simulink model "lab2p2"  (R2022a)
settings: Solver=VariableStepAuto  StartTime=0.0  StopTime=20  RelTol=1e-3
settings Model: Creator=tylergs2  LastModifiedBy=tylergs2

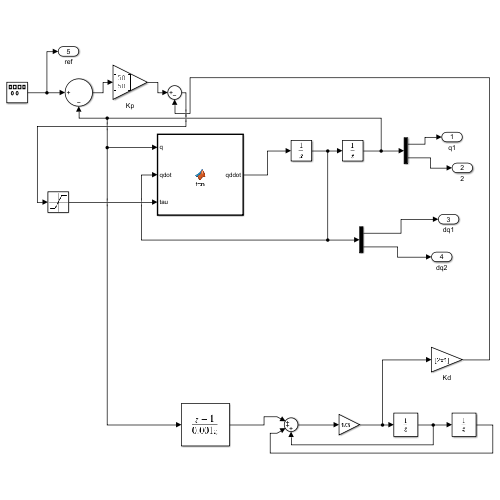
[thumbnail: Simulink's stored preview of the top-level diagram]
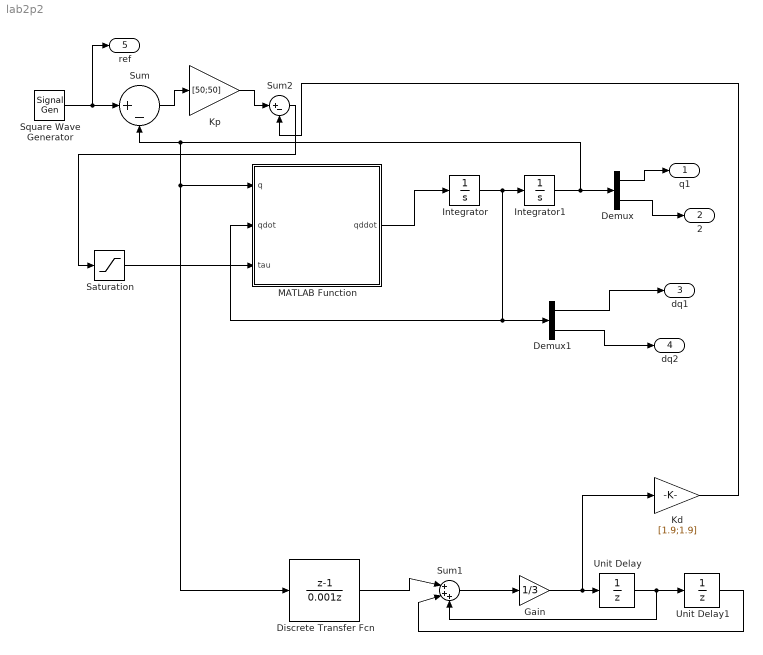
== system lab2p2 ==
  Demux : Demux  Outputs=2
  Demux1 : Demux  Outputs=2
  Discrete Transfer Fcn : DiscreteTransferFcn  Numerator="[1  -1]"  Denominator=[0.001 0]  SampleTime=0.001
  Gain : Gain  Gain=1/3
  Integrator : Integrator  InitialCondition=[0;0]
  Integrator1 : Integrator  InitialCondition=[0;0]
  Kd : Gain  Gain=[1.9;1.9]
  Kp : Gain  Gain=[50;50]
  MATLAB Function : MATLAB Function  TreatAsAtomicUnit=on
  Saturation : Saturate  UpperLimit=5  LowerLimit=-5
  Square Wave Generator : SignalGenerator  WaveForm=square  Amplitude=0.25  Frequency=0.25
  Sum : Sum  Inputs=|+-
  Sum1 : Sum  Inputs=|+++
  Sum2 : Sum  Inputs=|+-
  Unit Delay : UnitDelay  SampleTime=0.001  HasFrameUpgradeWarning=on
  Unit Delay1 : UnitDelay  SampleTime=0.001  HasFrameUpgradeWarning=on
  q1 : Outport
  2 : Outport  Port=2
  dq1 : Outport  Port=3
  dq2 : Outport  Port=4
  ref : Outport  Port=5
  wires:
  MATLAB Function/1(qddot) -> Integrator/1
  Integrator/1 -> Demux1/1, MATLAB Function/2(qdot), Integrator1/1
  Sum/1 -> Kp/1
  Discrete Transfer Fcn/1 -> Sum1/1
  Unit Delay1/1 -> Sum1/2
  Integrator1/1 -> Sum/2, Discrete Transfer Fcn/1, MATLAB Function/1(q), Demux/1
  Unit Delay/1 -> Sum1/3, Unit Delay1/1
  Gain/1 -> Kd/1, Unit Delay/1
  Sum1/1 -> Gain/1
  Kp/1 -> Sum2/1
  Kd/1 -> Sum2/2
  Square Wave Generator/1 -> ref/1, Sum/1
  Demux/1 -> q1/1
  Demux/2 -> 2/1
  Demux1/1 -> dq1/1
  Demux1/2 -> dq2/1
  Sum2/1 -> Saturation/1
  Saturation/1 -> MATLAB Function/3(tau)

== matlab function lab2p2/MATLAB Function ==
  data: q input; qddot output; qdot input; tau input
function qddot = fcn(q, qdot, tau)

g = 9.81;

p = [0.03; 0.0128; 0.0076; 0.0753; 0.0298];
D = [p(1), -p(3)*sin(q(2)-q(1)); -p(3)*sin(q(2)-q(1)), p(2)];
C = [0, -p(3)*cos(q(2)-q(1))*qdot(2); p(3)*cos(q(2)-q(1))*qdot(1), 0];
G = [-p(4)*g*sin(q(1)); -p(5)*g*cos(q(2))];

qddot = inv(D)*(tau - C*qdot - G);
